simulink subsystem "OcvBasedSocCalc_Subsys"  (R2025b)
settings: Solver=VariableStepAuto  StartTime=0.0  StopTime=10.0  RelTol=1e-3
undefined symbols (not defined in the file): KaSoc_degC_tempLut, KaSoc_frc_socLut, KaSoc_V_ocvLut
settings Model: Creator=Niharika  LastModifiedBy=Niharika
settings OptimizationCC: ReuseModelBlockBuffer=off
settings RTWCC: GPUComputeCapability=3.5

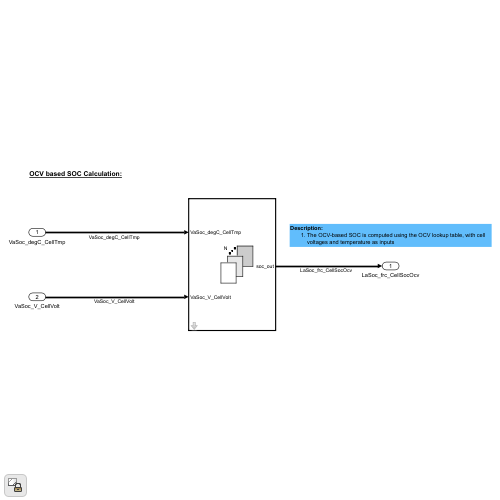
[thumbnail: Simulink's stored preview of the top-level diagram]
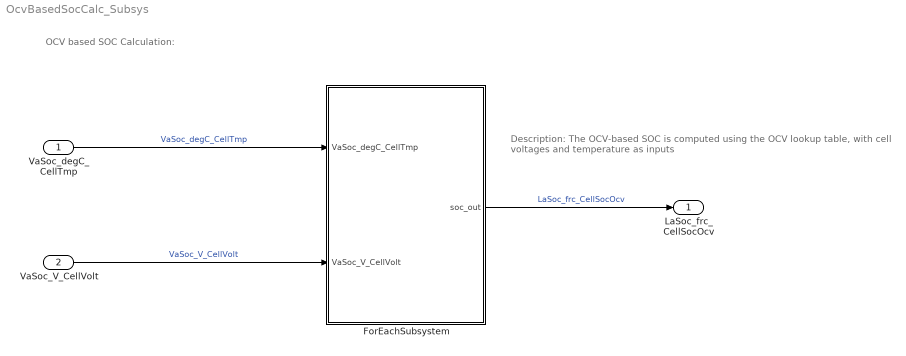
== system OcvBasedSocCalc_Subsys ==
  note: OCV based SOC Calculation:
  note: Description:
      | The OCV-based SOC is computed using the OCV lookup table, with cell voltages and temperature as inputs
  VaSoc_degC_CellTmp : Inport
  VaSoc_V_CellVolt : Inport  Port=2
  ForEachSubsystem : Subsystem  TreatAsAtomicUnit=on  mask{Temp_bp=KaSoc_degC_tempLut, SOC_bp=KaSoc_frc_socLut, OCV_bp=KaSoc_V_ocvLut}
  LaSoc_frc_CellSocOcv : Outport
  wires:
  VaSoc_degC_CellTmp/1 -> ForEachSubsystem/1(VaSoc_degC_CellTmp)  "VaSoc_degC_CellTmp"
  VaSoc_V_CellVolt/1 -> ForEachSubsystem/2(VaSoc_V_CellVolt)  "VaSoc_V_CellVolt"
  ForEachSubsystem/1(soc_out) -> LaSoc_frc_CellSocOcv/1  "LaSoc_frc_CellSocOcv"

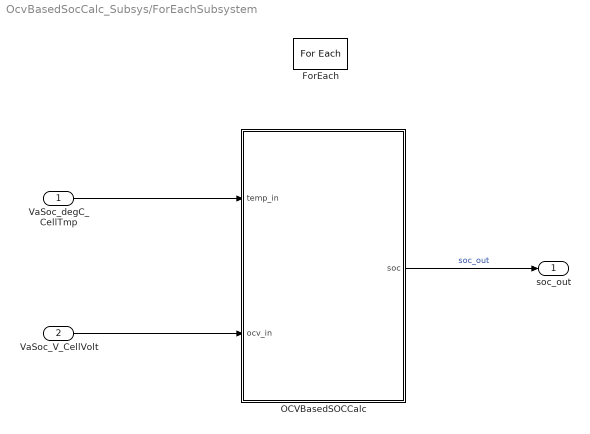
== system OcvBasedSocCalc_Subsys/ForEachSubsystem ==
  VaSoc_degC_CellTmp : Inport  Partition=on  PartitionDimension=1  PartitionWidth=1  PartitionOffset=0
  VaSoc_V_CellVolt : Inport  Port=2  Partition=on  PartitionDimension=1  PartitionWidth=1  PartitionOffset=0
  ForEach : ForEach  DisableCoverage=on  IterateSubsysMaskParameter=off,off,off
  OCVBasedSOCCalc : MATLAB Function  TreatAsAtomicUnit=on
      settings: RTWSystemCode=Inline
  soc_out : Outport  ConcatenationDimension=1
  wires:
  OCVBasedSOCCalc/1(soc) -> soc_out/1  "soc_out"
  VaSoc_V_CellVolt/1 -> OCVBasedSOCCalc/2(ocv_in)
  VaSoc_degC_CellTmp/1 -> OCVBasedSOCCalc/1(temp_in)

== matlab function OcvBasedSocCalc_Subsys/ForEachSubsystem/OCVBasedSOCCalc ==
  data: temp_in input size=[1 1]; soc output size=[1 1]; ocv_in input size=[1 1]; Temp_bp parameter double; SOC_bp parameter double; OCV_bp parameter double
%#codegen
function soc = OcvBasedSocLookupScalar(temp_in, ocv_in, Temp_bp, SOC_bp, OCV_bp)
    % Minimal-change scalar OCV+Temp SOC lookup suitable for For-Each subsystem.

    % numeric types
    temperature = double(temp_in);
    voltage     = double(ocv_in);

    Temp_bp = double(Temp_bp(:)');   % 1xM
    SOC_bp  = double(SOC_bp(:));     % Kx1
    OCV_bp  = double(OCV_bp);        % KxM

    % integer sizes for indexing (codegen-safe)
    numTemp_i = int32(length(Temp_bp));
    numSOC_i  = int32(length(SOC_bp));

    % thresholds (double)
    TEMPERATURE_EPS = 1e-6;
    VOLTAGE_EPS     = 1e-6;

    % ===============================
    % Temperature clamp + index find
    % ===============================
    if temperature <= Temp_bp(1)
        tempIndex = int32(1);
        tempFrac  = 0.0;

    elseif temperature >= Temp_bp(double(numTemp_i))
        tempIndex = numTemp_i - int32(1);
        tempFrac  = 1.0;

    else
        % default integer index
        tempIndex = int32(1);
        for tempIdx = int32(1):int32(numTemp_i - 1)
            if temperature <= Temp_bp(tempIdx + int32(1))
                tempIndex = tempIdx;
                break;
            end
        end

        % safety clamp
        if tempIndex < int32(1)
            tempIndex = int32(1);
        elseif tempIndex > (numTemp_i - int32(1))
            tempIndex = numTemp_i - int32(1);
        end

        T0 = Temp_bp(tempIndex);
        T1 = Temp_bp(tempIndex + int32(1));
        deltaT = T1 - T0;

        if deltaT > TEMPERATURE_EPS
            tempFrac = (temperature - T0) / deltaT;
            if tempFrac < 0.0
                tempFrac = 0.0;
            elseif tempFrac > 1.0
                tempFrac = 1.0;
            end
        else
            tempFrac = 0.0;
        end
    end

    % ===============================
    % SOC lookup at T0
    % ===============================
    ocvRow0 = OCV_bp(:, tempIndex);

    if voltage <= ocvRow0(1)
        socT0 = SOC_bp(1);

    elseif voltage >= ocvRow0(double(numSOC_i))
        socT0 = SOC_bp(double(numSOC_i));

    else
        socIdx = int32(1);
        for idxSOC = int32(1):int32(numSOC_i - 1)
            if voltage <= ocvRow0(idxSOC + int32(1))
                socIdx = idxSOC;
                break;
            end
        end

        if socIdx < int32(1)
            socIdx = int32(1);
        elseif socIdx > (numSOC_i - int32(1))
            socIdx = numSOC_i - int32(1);
        end

        v0 = ocvRow0(socIdx);
        v1 = ocvRow0(socIdx + int32(1));
        s0 = SOC_bp(socIdx);
        s1 = SOC_bp(socIdx + int32(1));

        dv = v1 - v0;

        if dv == 0 || (dv*dv < VOLTAGE_EPS * VOLTAGE_EPS)
            % flat or near-flat → midpoint
            socT0 = 0.5 * (s0 + s1);
        else
            frac = (voltage - v0) / dv;
            socT0 = s0 + frac * (s1 - s0);
        end
    end

    % ===============================
    % SOC lookup at T1
    % ===============================
    ocvRow1 = OCV_bp(:, tempIndex + int32(1));

    if voltage <= ocvRow1(1)
        socT1 = SOC_bp(1);

    elseif voltage >= ocvRow1(double(numSOC_i))
        socT1 = SOC_bp(double(numSOC_i));

    else
        socIdx2 = int32(1);
        for idxSOC = int32(1):int32(numSOC_i - 1)
            if voltage <= ocvRow1(idxSOC + int32(1))
                socIdx2 = idxSOC;
                break;
            end
        end

        if socIdx2 < int32(1)
            socIdx2 = int32(1);
        elseif socIdx2 > (numSOC_i - int32(1))
            socIdx2 = numSOC_i - int32(1);
        end

        v0 = ocvRow1(socIdx2);
        v1 = ocvRow1(socIdx2 + int32(1));
        s0 = SOC_bp(socIdx2);
        s1 = SOC_bp(socIdx2 + int32(1));

        dv2 = v1 - v0;

        if dv2 == 0 || (dv2*dv2 < VOLTAGE_EPS * VOLTAGE_EPS)
            socT1 = 0.5 * (s0 + s1);
        else
            frac2 = (voltage - v0) / dv2;
            socT1 = s0 + frac2 * (s1 - s0);
        end
    end

    % ===============================
    % Final bilinear interpolation
    % ===============================
    soc_d = socT0 + tempFrac * (socT1 - socT0);

    if soc_d < 0
        soc_d = 0;
    elseif soc_d > 1
        soc_d = 1;
    end

    soc = single(soc_d);
end
